simulink model "path_following_PID"  (R2022a)
settings: Solver=VariableStepAuto  StartTime=0.0  StopTime=10  RelTol=1e-3
undefined symbols (not defined in the file or in its folder): curvature, direction, gradbp, psi_o, thetaRefs, xRef2s, yRef2s
libraries: slpidlib x2, simulink x2, simulink_extras x1
settings Model: Creator=andreagottardini  LastModifiedBy=andreagottardini

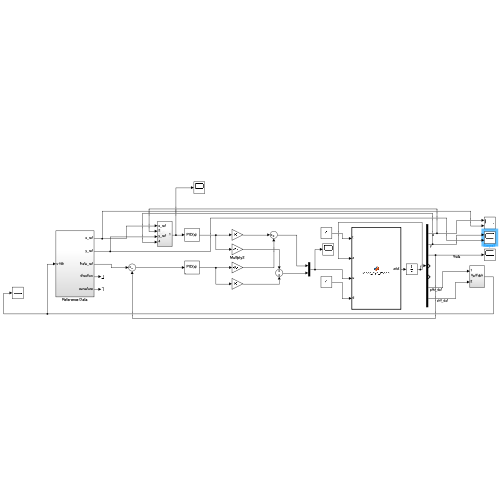
[thumbnail: Simulink's stored preview of the top-level diagram]
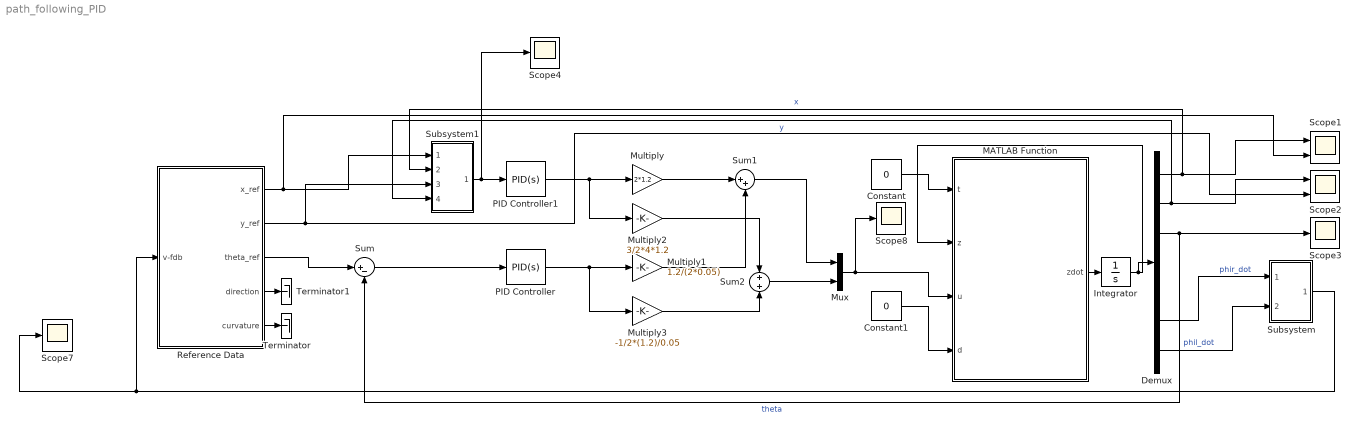
== system path_following_PID ==
  Constant : Constant  Value=0
  Constant1 : Constant  Value=0
  Demux : Demux  Outputs=7
  Integrator : Integrator  InitialCondition=[-33.600000000000000;-1.100000000000000;0;0;0;0;0]
  MATLAB Function : MATLAB Function  TreatAsAtomicUnit=on
  Multiply : Gain  Gain=2*1.2
  Multiply1 : Gain  Gain=1.2/(2*0.05)
  Multiply2 : Gain  Gain=3/2*4*1.2
  Multiply3 : Gain  Gain=-1/2*(1.2)/0.05
  Mux : Mux  Inputs=2
  PID Controller : slpidlib/PID Controller  Controller=PID  Form=Parallel  TimeDomain=Continuous-time  UseExternalTs=off  SampleTime=-1  IntegratorMethod=Forward Euler  FilterMethod=Forward Euler  ControllerParametersSource=internal  P=0.0021057  I=0.0037144  UseKiTs=off  D=0.00011785  N=30  UseFilter=on  TunerSelectOption=Frequency Response Based  InitialConditionSource=internal  InitialConditionForIntegrator=0  InitialConditionForFilter=0  DifferentiatorICPrevScaledInput=0  ExternalReset=none  TrackingMode=off  Kt=1  LimitOutput=off  SatLimitsSource=internal  UpperSaturationLimit=inf  LowerSaturationLimit=-inf  LinearizeAsGain=on  AntiWindupMode=none  Kb=1  POutMin=[]  POutMax=[]  IOutMin=[]  IOutMax=[]  DOutMin=[]  DOutMax=[]  NOutMin=[]  NOutMax=[]  SumOutMin=[]  SumOutMax=[]  SaturationOutMin=[]  SaturationOutMax=[]  PParamMin=[]  PParamMax=[]  IParamMin=[]  IParamMax=[]  DParamMin=[]  DParamMax=[]  NParamMin=[]  NParamMax=[]  KbParamMin=[]  KbParamMax=[]  KtParamMin=[]  KtParamMax=[]  KbOutMin=[]  KbOutMax=[]  KtOutMin=[]  KtOutMax=[]  IntegratorOutMin=[]  IntegratorOutMax=[]  FilterOutMin=[]  FilterOutMax=[]  SumI1OutMin=[]  SumI1OutMax=[]  SumI2OutMin=[]  SumI2OutMax=[]  SumI3OutMin=[]  SumI3OutMax=[]  SumI4OutMin=[]  SumI4OutMax=[]  SumDOutMin=[]  SumDOutMax=[]  DifferentiatorOutMin=[]  DifferentiatorOutMax=[]  FilterDiffOutCoefMin=[]  FilterDiffOutCoefMax=[]  ReciprocalOutMin=[]  ReciprocalOutMax=[]  SumDenOutMin=[]  SumDenOutMax=[]  SumNumOutMin=[]  SumNumOutMax=[]  DivideOutMin=[]  DivideOutMax=[]  UdiffTsProdOutMin=[]  UdiffTsProdOutMax=[]  NTsProdOutMin=[]  NTsProdOutMax=[]  UintegralTsProdOutMin=[]  UintegralTsProdOutMax=[]  UngainTsProdOutMin=[]  UngainTsProdOutMax=[]  IntegratorContinuousStateAttributes=''  IntegratorStateMustResolveToSignalObject=off  IntegratorRTWStateStorageClass=Auto  FilterContinuousStateAttributes=''  FilterStateMustResolveToSignalObject=off  FilterRTWStateStorageClass=Auto  ParallelPVariant=InternalParameters  IdealPVariant=Disabled  IVariant=InternalParameters  DVariant=InternalParameters  IntegratorVariant=Continuous  SatVariant=Disabled  AWVariant=Passthrough  PCopyVariant=Disabled  TRVariant=Disabled  FdbkBlocksVariant=Forward  IdealPFdbkVariant=Disabled  SatFdbkVariant=Disabled  DerivativeFilterVariant=ContFilter  NVariant=InternalParameters  NCopyVariant=Disabled  FilterICVariant=InternalICsFilter  IntegratorICVariant=InternalICs  ExternalResetVariant=Disabled  TRSumVariant=Passthrough  SumFdbkVariant=Disabled  SumVariant=Sum_PID  TsampFilterVariant=InternalTs  TsampNgainVariant=Passthrough  TsampIntegralVariant=Passthrough  ExternalSaturationOutDataTypeStr=Inherit: Same as second input  aMode=0
  PID Controller1 : slpidlib/PID Controller  Controller=PID  Form=Parallel  TimeDomain=Continuous-time  UseExternalTs=off  SampleTime=-1  IntegratorMethod=Forward Euler  FilterMethod=Forward Euler  ControllerParametersSource=internal  P=0  I=-12.1563  UseKiTs=off  D=-0.10685  N=300  UseFilter=on  TunerSelectOption=Frequency Response Based  InitialConditionSource=internal  InitialConditionForIntegrator=0  InitialConditionForFilter=0  DifferentiatorICPrevScaledInput=0  ExternalReset=none  TrackingMode=off  Kt=1  LimitOutput=off  SatLimitsSource=internal  UpperSaturationLimit=inf  LowerSaturationLimit=-inf  LinearizeAsGain=on  AntiWindupMode=none  Kb=1  POutMin=[]  POutMax=[]  IOutMin=[]  IOutMax=[]  DOutMin=[]  DOutMax=[]  NOutMin=[]  NOutMax=[]  SumOutMin=[]  SumOutMax=[]  SaturationOutMin=[]  SaturationOutMax=[]  PParamMin=[]  PParamMax=[]  IParamMin=[]  IParamMax=[]  DParamMin=[]  DParamMax=[]  NParamMin=[]  NParamMax=[]  KbParamMin=[]  KbParamMax=[]  KtParamMin=[]  KtParamMax=[]  KbOutMin=[]  KbOutMax=[]  KtOutMin=[]  KtOutMax=[]  IntegratorOutMin=[]  IntegratorOutMax=[]  FilterOutMin=[]  FilterOutMax=[]  SumI1OutMin=[]  SumI1OutMax=[]  SumI2OutMin=[]  SumI2OutMax=[]  SumI3OutMin=[]  SumI3OutMax=[]  SumI4OutMin=[]  SumI4OutMax=[]  SumDOutMin=[]  SumDOutMax=[]  DifferentiatorOutMin=[]  DifferentiatorOutMax=[]  FilterDiffOutCoefMin=[]  FilterDiffOutCoefMax=[]  ReciprocalOutMin=[]  ReciprocalOutMax=[]  SumDenOutMin=[]  SumDenOutMax=[]  SumNumOutMin=[]  SumNumOutMax=[]  DivideOutMin=[]  DivideOutMax=[]  UdiffTsProdOutMin=[]  UdiffTsProdOutMax=[]  NTsProdOutMin=[]  NTsProdOutMax=[]  UintegralTsProdOutMin=[]  UintegralTsProdOutMax=[]  UngainTsProdOutMin=[]  UngainTsProdOutMax=[]  IntegratorContinuousStateAttributes=''  IntegratorStateMustResolveToSignalObject=off  IntegratorRTWStateStorageClass=Auto  FilterContinuousStateAttributes=''  FilterStateMustResolveToSignalObject=off  FilterRTWStateStorageClass=Auto  ParallelPVariant=InternalParameters  IdealPVariant=Disabled  IVariant=InternalParameters  DVariant=InternalParameters  IntegratorVariant=Continuous  SatVariant=Disabled  AWVariant=Passthrough  PCopyVariant=Disabled  TRVariant=Disabled  FdbkBlocksVariant=Forward  IdealPFdbkVariant=Disabled  SatFdbkVariant=Disabled  DerivativeFilterVariant=ContFilter  NVariant=InternalParameters  NCopyVariant=Disabled  FilterICVariant=InternalICsFilter  IntegratorICVariant=InternalICs  ExternalResetVariant=Disabled  TRSumVariant=Passthrough  SumFdbkVariant=Disabled  SumVariant=Sum_PID  TsampFilterVariant=InternalTs  TsampNgainVariant=Passthrough  TsampIntegralVariant=Passthrough  ExternalSaturationOutDataTypeStr=Inherit: Same as second input  aMode=0
  Reference Data : Subsystem  VariantControl=Stanley
  Scope1 : Scope  NumInputPorts=2
  Scope2 : Scope  NumInputPorts=2
  Scope{3..4,7..8} (4 alike) : Scope
  Subsystem : Subsystem
  Subsystem1 : Subsystem
  Sum : Sum  Inputs=|+-
  Sum1 : Sum  Inputs=|++
  Sum2 : Sum
  Terminator : Terminator
  Terminator1 : Terminator
  wires:
  Constant/1 -> MATLAB Function/1(t)
  Constant1/1 -> MATLAB Function/4(d)
  Subsystem/1(VelFdbk) -> Reference Data/1(v-fdb), Scope7/1
  Reference Data/3(theta_ref) -> Sum/1
  Demux/3 -> Sum/2, Scope3/1  "theta"
  Reference Data/2(y_ref) -> Scope2/2, Subsystem1/3(y_ref)
  Demux/1 -> Scope1/1, Subsystem1/2(In2)  "x"
  Demux/2 -> Subsystem1/4(In4), Scope2/1  "y"
  Multiply/1 -> Sum1/1
  Multiply1/1 -> Sum1/2
  Sum1/1 -> Mux/1
  Mux/1 -> Scope8/1, MATLAB Function/3(u)
  Multiply2/1 -> Sum2/1
  Multiply3/1 -> Sum2/2
  Sum2/1 -> Mux/2
  Demux/6 -> Subsystem/1(In1)  "phir_dot"
  Demux/7 -> Subsystem/2(In2)  "phil_dot"
  Integrator/1 -> MATLAB Function/2(z), Demux/1
  Reference Data/4(direction) -> Terminator1/1
  Reference Data/5(curvature) -> Terminator/1
  Reference Data/1(x_ref) -> Scope1/2, Subsystem1/1(x_ref)
  MATLAB Function/1(zdot) -> Integrator/1
  PID Controller/1 -> Multiply3/1, Multiply1/1
  Sum/1 -> PID Controller/1
  PID Controller1/1 -> Multiply2/1, Multiply/1
  Subsystem1/1(Out1) -> PID Controller1/1, Scope4/1

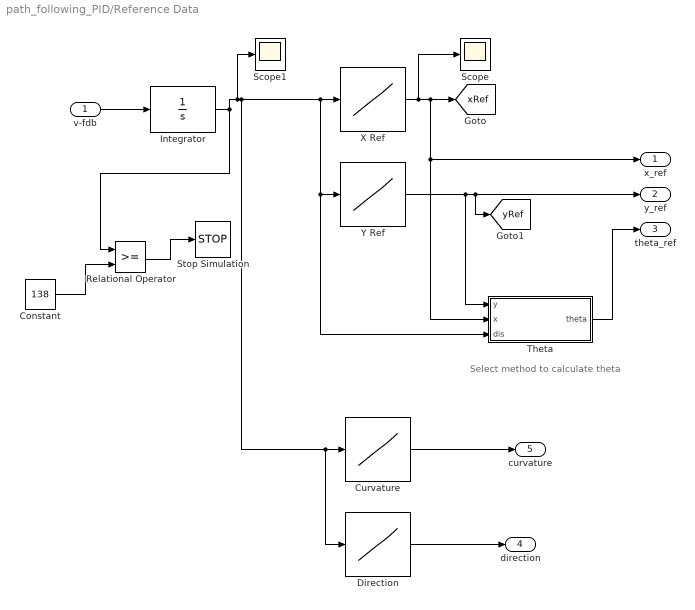
== system path_following_PID/Reference Data ==
  note: Select method to calculate theta
  v-fdb : Inport
  Constant : Constant  Value=138
  Curvature : Lookup_n-D  NumberOfTableDimensions=1  BreakpointsForDimension1=gradbp  Table=curvature  InternalRulePriority=Speed  RndMeth=Simplest
  Direction : Lookup_n-D  NumberOfTableDimensions=1  BreakpointsForDimension1=gradbp  Table=direction  InternalRulePriority=Speed  RndMeth=Simplest
  Integrator : Integrator
  Relational Operator : RelationalOperator  OutDataTypeStr=boolean  RndMeth=Simplest  InputSameDT=off
  Scope : Scope
  Scope1 : Scope
  Stop Simulation : Stop
  Theta : Subsystem  Variant=on  VariantControlMode=label  LabelModeActiveChoice=thetaSimulinkBlock
  X Ref : Lookup_n-D  NumberOfTableDimensions=1  BreakpointsForDimension1=gradbp  Table=xRef2s  InternalRulePriority=Speed  RndMeth=Simplest
  Y Ref : Lookup_n-D  NumberOfTableDimensions=1  BreakpointsForDimension1=gradbp  Table=yRef2s  InternalRulePriority=Speed  RndMeth=Simplest
  x_ref : Outport
  y_ref : Outport  Port=2
  theta_ref : Outport  Port=3
  direction : Outport  Port=4
  curvature : Outport  Port=5
  tag scope: xRef=global, yRef=global
  wires:
  Direction/1 -> direction/1
  Curvature/1 -> curvature/1
  Y Ref/1 -> Theta/1(y), y_ref/1, [yRef]
  X Ref/1 -> Scope/1, x_ref/1, Theta/2(x), [xRef]
  Integrator/1 -> Scope1/1, Curvature/1, Direction/1, Theta/3(dis), Y Ref/1, X Ref/1, Relational Operator/1
  Theta/1(theta) -> theta_ref/1
  v-fdb/1 -> Integrator/1
  Relational Operator/1 -> Stop Simulation/1
  Constant/1 -> Relational Operator/2

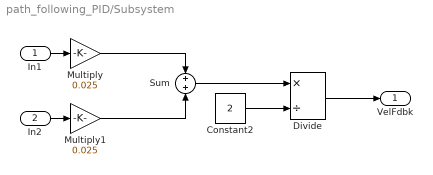
== system path_following_PID/Subsystem ==
  In1 : Inport
  In2 : Inport  Port=2
  Constant2 : Constant  Value=2
  Divide : Product  Inputs=*/
  Multiply : Gain  Gain=0.025
  Multiply1 : Gain  Gain=0.025
  Sum : Sum  Inputs=+|+
  VelFdbk : Outport
  wires:
  Constant2/1 -> Divide/2
  Sum/1 -> Divide/1
  Multiply/1 -> Sum/1
  Divide/1 -> VelFdbk/1
  In1/1 -> Multiply/1
  In2/1 -> Multiply1/1
  Multiply1/1 -> Sum/2

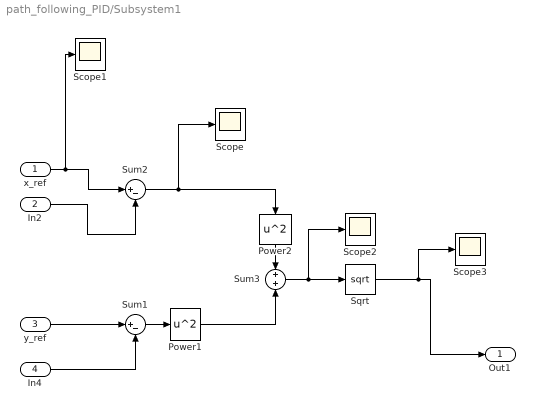
== system path_following_PID/Subsystem1 ==
  x_ref : Inport
  In2 : Inport  Port=2
  y_ref : Inport  Port=3
  In4 : Inport  Port=4
  Power1 : Math  Operator=square
  Power2 : Math  Operator=square
  Scope{,1..3} (4 alike) : Scope
  Sqrt : Sqrt
  Sum1 : Sum  Inputs=|+-
  Sum2 : Sum  Inputs=|+-
  Sum3 : Sum
  Out1 : Outport
  wires:
  Sqrt/1 -> Scope3/1, Out1/1
  y_ref/1 -> Sum1/1
  Sum3/1 -> Scope2/1, Sqrt/1
  In2/1 -> Sum2/2
  x_ref/1 -> Scope1/1, Sum2/1
  In4/1 -> Sum1/2
  Sum1/1 -> Power1/1
  Power1/1 -> Sum3/2
  Sum2/1 -> Scope/1, Power2/1
  Power2/1 -> Sum3/1

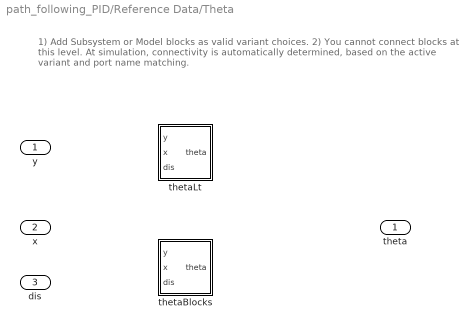
== system path_following_PID/Reference Data/Theta ==
  note: 1) Add Subsystem or Model blocks as valid variant choices.
      | 2) You cannot connect blocks at this level. At simulation, connectivity is automatically
      | determined, based on the active variant and port name matching.
  y : Inport
  x : Inport  Port=2
  dis : Inport  Port=3
  thetaBlocks : Subsystem  VariantControl=thetaSimulinkBlock
  thetaLt : Subsystem  VariantControl=thetaLookUpTable
  theta : Outport

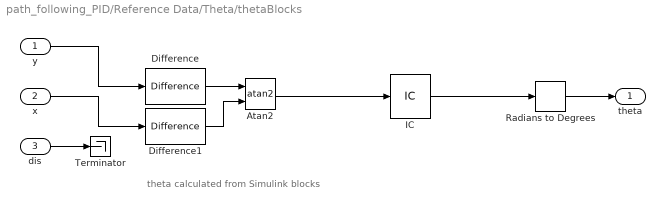
== system path_following_PID/Reference Data/Theta/thetaBlocks ==
  note: theta calculated from Simulink blocks
  y : Inport
  x : Inport  Port=2
  dis : Inport  Port=3
  Atan2 : Trigonometry  Operator=atan2  ApproximationMethod=CORDIC
  Difference : simulink/Discrete/Difference  ICPrevInput=0.0  OutMin=[]  OutMax=[]  OutDataType=fixdt(1, 16)  OutScaling=2^-10  DoSatur=off
  Difference1 : simulink/Discrete/Difference  ICPrevInput=0.0  OutMin=[]  OutMax=[]  OutDataType=fixdt(1, 16)  OutScaling=2^-10  DoSatur=off
  IC : InitialCondition  Value=psi_o
  Radians to Degrees : simulink_extras/Transformations/Radians to Degrees
  Terminator : Terminator
  theta : Outport
  wires:
  IC/1 -> Radians to Degrees/1
  Atan2/1 -> IC/1
  dis/1 -> Terminator/1
  x/1 -> Difference1/1
  y/1 -> Difference/1
  Radians to Degrees/1 -> theta/1
  Difference/1 -> Atan2/1
  Difference1/1 -> Atan2/2

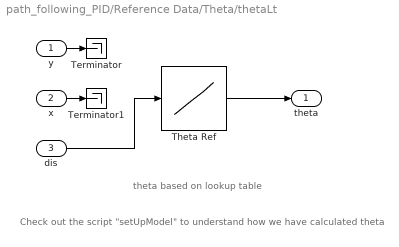
== system path_following_PID/Reference Data/Theta/thetaLt ==
  note: Check out the script "setUpModel" to understand how we have calculated theta
  note: theta based on lookup table
  y : Inport
  x : Inport  Port=2
  dis : Inport  Port=3
  Terminator : Terminator
  Terminator1 : Terminator
  Theta Ref : Lookup_n-D  NumberOfTableDimensions=1  BreakpointsForDimension1=gradbp  Table=thetaRefs  InternalRulePriority=Speed  RndMeth=Simplest
  theta : Outport
  wires:
  Theta Ref/1 -> theta/1
  dis/1 -> Theta Ref/1
  x/1 -> Terminator1/1
  y/1 -> Terminator/1

== matlab function path_following_PID/MATLAB Function ==
  data: t input; z input; u input; zdot output; d input
function zdot=robot_dyn_model(t,z,u,d)

%% Read parameters, states and inputs

% Parameters
% Ic      =       th(1,1);     %
% Iw      =       th(2,1);     % 
% d       =       th(3,1);     % 
% mw      =       th(4,1);     % 
% mc      =       th(5,1);     % 
% Im      =       th(6,1);     % 
% R       =       th(7,1);     % 
% L       =       th(8,1);     % 

 Ic      =       1;     %
 Iw      =       0.1;     % 
 d       =       0.05;     % 
 mw      =       0.1;     % 
 mc      =       1;     % 
 Im      =       0.1;     % 
 R       =       0.025;     % 
 L       =       0.05;

mT = mc+2*mw;
I = Ic+mc*d^2+2*mw*L^2+2*Im;


% States
xa                  =       z(1,1);    % inertial X position (m)
ya                  =       z(2,1);    % inertial Y position (m)
theta               =       z(3,1);    % body orientation - yaw angle(rad)
phir                =       z(4,1);    % angular displacement right wheel (rad)
phil                =       z(5,1);    % angular displacement left wheel (rad)
phir_dot            =       z(6,1);    % angular velocity right wheel (rad/s)    
phil_dot            =       z(7,1);    % angular velocity left wheel (rad/s)



% Additional paramaeters
cth = cos(theta);
sth = sin(theta);

lam = [-sth     cth     0;
        cth     sth     L;
        cth     sth     -L];

b = inv(lam)*[0; R*phir_dot; R*phil_dot];

xa_dot      =    b(1,1);
ya_dot      =    b(2,1);
theta_dot   =    b(3,1);




% Inputs
taur      =       u(1,1);     % driving/braking torque right wheel (N*m)
taul      =       u(2,1);     % driving/braking torque left wheel (N*m)


%% Matrices


S = [R/(2*L)*(L*cth-d*sth) R/(2*L)*(L*cth+d*sth);
     R/(2*L)*(L*sth+d*cth) R/(2*L)*(L*sth-d*cth);
     R/(2*L)               -R/(2*L)             ;
     1                      0                   ;
     0                      1];


M_bar = [Iw+R^2/(4*L^2)*(mT*L^2+I)          R^2/(4*L^2)*(mT*L^2-I); 
        R^2/(4*L^2)*(mT*L^2-I)              Iw+R^2/(4*L^2)*(mT*L^2+I)];

V_bar = [0                              R^2/(2*L)*mc*d*theta_dot;
        -R^2/(2*L)*mc*d*theta_dot               0];



% Model equations

zdot = zeros(7,1);

zdot = [S*z(6:7,1); zeros(2,1)] + [zeros(5,2); eye(2)]*inv(M_bar)*(u-V_bar*z(6:7,1));
